simulink model "nn_gensim"  (R2016a)
settings: Solver=VariableStepAuto  StartTime=0.0  StopTime=10.0  RelTol=1e-3
libraries: neural x66
(part 2 of 2)

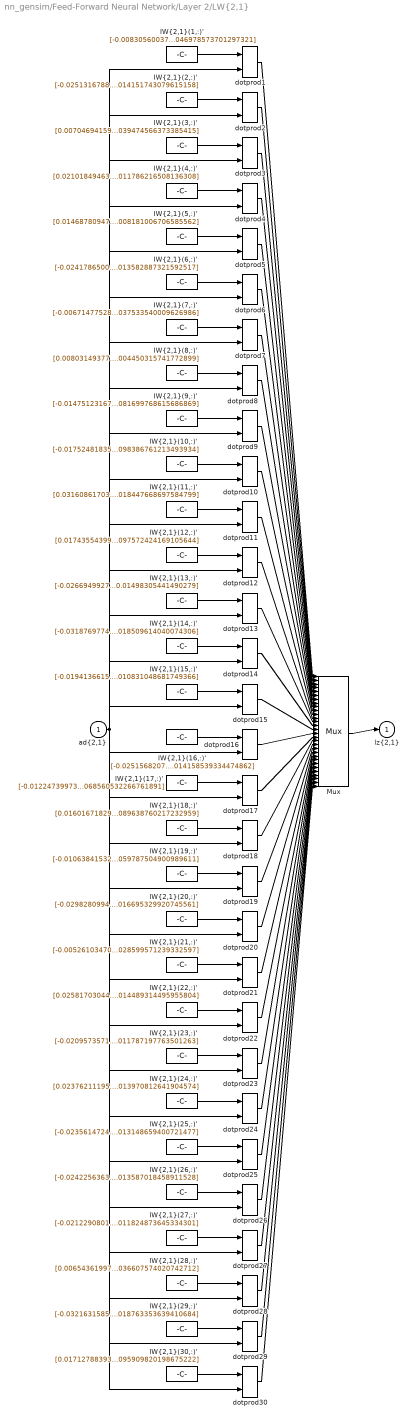
== system nn_gensim/Feed-Forward Neural Network/Layer 2/LW{2,1} ==
  "ad{2,1}" : Inport  PortDimensions=30
      mask Display: e = 0.06;c1 = [120 230 180]/255;c2 = ([120 230 180]+0)/(256+128);c3 = ([120 230 180]+128)/(256+128);patch([0 1 1 0],[0 0 1 1],c1);patch([0 1 1 1-e 1-e 0+e],[0 0 1 1-e 0+e 0+e],c2);patch([0 0 1 1-e 0+e 0+e],[0 1 1 1-e 1-e 0+e],c3);plot([0 1 1 0 0],[0 0 1 1 0]);
  "IW{2,1}(1,:)'" : Constant  Value=[-0.0083056003756890144;0.019113962537947015;-0.0089497074294720546;-0.0098923334864796566;-0.023988299220988073;-0.0018485816845016079;-0.0059618452261974968;0.0069988362336697064;0.036667021342056919;0.016526862034832963;0.030193069855730826;-0.0047630507834777354;-0.018046869018482389;-0.0057026826950931355;0.037752079200427259;0.016557695091664312;0.013106033602432574;-0.019925230456181005;0.039680560899078204;0.025432917279803999;0.00072297603107219274;-0.019455142955335462;-0.01509695277684032;-0.013561420755406835;-0.00075464259463946162;-0.017391870248462917;0.010751916691427063;-0.0050629731985845586;-0.00071487359349162725;-0.0046978573701297321]
      mask Display: e = 0.06;c1 = [120 150 230]/255;c2 = ([120 150 230]+0)/383;c3 = ([120 150 230]+128)/383;patch([0 1 1 0],[0 0 1 1],c1);patch([0 1 1 1-e 1-e 0+e],[0 0 1 1-e 0+e 0+e],c2);patch([0 0 1 1-e 0+e 0+e],[0 1 1 1-e 1-e 0+e],c3);plot([0 1 1 0 0],[0 0 1 1 0]);disp('weights');
  "IW{2,1}(10,:)'" : Constant  Value=[-0.017524818358626806;0.040334814474458656;-0.018584934026375351;-0.020997681047963575;-0.050780548941037972;-0.0034476905494047519;-0.012647174473932836;0.015275522704802792;0.078915212404200449;0.034766129023966738;0.064914340733501982;-0.010010282680391055;-0.038131544108099727;-0.01206243778923099;0.084105228253449155;0.034674216527232619;0.02736829412730514;-0.042075183943914629;0.085704139620146225;0.053900839834691287;0.00099753662040386764;-0.042854177306582489;-0.031996880085286478;-0.028247287853701203;-0.001588847763167444;-0.036339886541172157;0.02264214185105046;-0.01060981341310595;-0.0013587789640045617;-0.0098386761213493934]
      mask Display: e = 0.06;c1 = [120 150 230]/255;c2 = ([120 150 230]+0)/383;c3 = ([120 150 230]+128)/383;patch([0 1 1 0],[0 0 1 1],c1);patch([0 1 1 1-e 1-e 0+e],[0 0 1 1-e 0+e 0+e],c2);patch([0 0 1 1-e 0+e 0+e],[0 1 1 1-e 1-e 0+e],c3);plot([0 1 1 0 0],[0 0 1 1 0]);disp('weights');
  "IW{2,1}(11,:)'" : Constant  Value=[0.031608617033696336;-0.072894856159988572;0.032497541258948992;0.037028062293751475;0.095065968405568177;-0.0025854679662332446;0.022672609607487734;-0.041977003552746424;-0.16800834621404154;-0.060763296536032602;-0.12889957814084452;0.017891408952875096;0.06899010013800265;0.021490887029687971;-0.19237659860623346;-0.059468024825016903;-0.047814292076542045;0.075198049752529444;-0.1858796335369855;-0.10190145864029221;0.0063443741930746611;0.10313747460923257;0.054986646969208179;0.047198965962547634;0.0029349224226672445;0.064302452214189551;-0.041238190569702141;0.019490075273115491;-0.00079340138722999178;0.018447668697584799]
      mask Display: e = 0.06;c1 = [120 150 230]/255;c2 = ([120 150 230]+0)/383;c3 = ([120 150 230]+128)/383;patch([0 1 1 0],[0 0 1 1],c1);patch([0 1 1 1-e 1-e 0+e],[0 0 1 1-e 0+e 0+e],c2);patch([0 0 1 1-e 0+e 0+e],[0 1 1 1-e 1-e 0+e],c3);plot([0 1 1 0 0],[0 0 1 1 0]);disp('weights');
  "IW{2,1}(12,:)'" : Constant  Value=[0.017435543996330929;-0.040142341143420017;0.018474701322763559;0.020931966839192878;0.050465323426277402;0.0034269848078252287;0.012633810047245017;-0.015119790757508161;-0.078491892194480786;-0.034614559781884137;-0.064676958157261766;0.0099795662119423305;0.037936781443958942;0.01201366890879701;-0.083827652877886474;-0.034520744867777162;-0.027203928877341771;0.041896869180871113;-0.085215347287222645;-0.053599186633662151;-0.00091781479818617848;0.042664029462400249;0.031885742582713816;0.028118222040869573;0.0016132091520745346;0.036122832809355798;-0.022546412528904554;0.010549377908676376;0.0013479033309776211;0.0097572424169105644]
      mask Display: e = 0.06;c1 = [120 150 230]/255;c2 = ([120 150 230]+0)/383;c3 = ([120 150 230]+128)/383;patch([0 1 1 0],[0 0 1 1],c1);patch([0 1 1 1-e 1-e 0+e],[0 0 1 1-e 0+e 0+e],c2);patch([0 0 1 1-e 0+e 0+e],[0 1 1 1-e 1-e 0+e],c3);plot([0 1 1 0 0],[0 0 1 1 0]);disp('weights');
  "IW{2,1}(13,:)'" : Constant  Value=[-0.026694992742945192;0.061612330161735056;-0.027653274803672748;-0.03209017288048447;-0.078339461809738109;-0.0032984920599325039;-0.019280886778573432;0.026125586559889606;0.12672985074381135;0.05254292205453958;0.1028317373080775;-0.015138719899045418;-0.058465378962648439;-0.018410447742282243;0.1426089569060506;0.052051523127150716;0.04105910843020593;-0.064224935000000025;0.138707895630444;0.08350353784434883;-0.00030259207296238805;-0.07217030681977768;-0.048668504265280944;-0.041978413631100872;-0.0024148634335991151;-0.054664063752061842;0.034457407503966898;-0.016116981449881235;-0.0014601988631814827;-0.01498305441490279]
      mask Display: e = 0.06;c1 = [120 150 230]/255;c2 = ([120 150 230]+0)/383;c3 = ([120 150 230]+128)/383;patch([0 1 1 0],[0 0 1 1],c1);patch([0 1 1 1-e 1-e 0+e],[0 0 1 1-e 0+e 0+e],c2);patch([0 0 1 1-e 0+e 0+e],[0 1 1 1-e 1-e 0+e],c3);plot([0 1 1 0 0],[0 0 1 1 0]);disp('weights');
  "IW{2,1}(14,:)'" : Constant  Value=[-0.031876977425942685;0.073285499375244853;-0.032295188882699936;-0.037736257112251752;-0.095092447058463245;0.0019240694986817509;-0.022816584395266189;0.040823302705698998;0.16712898248422273;0.060936001349780548;0.12924032585515743;-0.018092945230880942;-0.0694696033517158;-0.021829863852450747;0.19349763967940106;0.059401581781717866;0.047644816424967033;-0.075452140330637518;0.18487501046910346;0.10189553984576843;-0.0055389784205687204;-0.10212528536332899;-0.055994220935609171;-0.047221755005684672;-0.0027621280402611013;-0.064064251531706889;0.041262423698454148;-0.019555242969875469;0.00034805824680751067;-0.018509614040074306]
      mask Display: e = 0.06;c1 = [120 150 230]/255;c2 = ([120 150 230]+0)/383;c3 = ([120 150 230]+128)/383;patch([0 1 1 0],[0 0 1 1],c1);patch([0 1 1 1-e 1-e 0+e],[0 0 1 1-e 0+e 0+e],c2);patch([0 0 1 1-e 0+e 0+e],[0 1 1 1-e 1-e 0+e],c3);plot([0 1 1 0 0],[0 0 1 1 0]);disp('weights');
  "IW{2,1}(15,:)'" : Constant  Value=[-0.019413661578074042;0.044673634539894612;-0.020394867098211009;-0.023348838301773287;-0.056280148408457936;-0.0036788192590742575;-0.014022602890496248;0.017013476590978686;0.087887652471076952;0.038469248573656904;0.072368779142843398;-0.01104288846513549;-0.042281634449772523;-0.013408340227602867;0.095064024539261799;0.038256301227484087;0.030197680839771299;-0.046633071114016482;0.095560722206547571;0.059748872737462252;0.00094440913626948127;-0.048078919304247077;-0.035576359111311552;-0.03112221349266709;-0.001759051666175712;-0.040014263931521771;0.02503986639519926;-0.011699415523057108;-0.0014869690523505858;-0.010831048681749366]
      mask Display: e = 0.06;c1 = [120 150 230]/255;c2 = ([120 150 230]+0)/383;c3 = ([120 150 230]+128)/383;patch([0 1 1 0],[0 0 1 1],c1);patch([0 1 1 1-e 1-e 0+e],[0 0 1 1-e 0+e 0+e],c2);patch([0 0 1 1-e 0+e 0+e],[0 1 1 1-e 1-e 0+e],c3);plot([0 1 1 0 0],[0 0 1 1 0]);disp('weights');
  "IW{2,1}(16,:)'" : Constant  Value=[-0.025156820762488812;0.058054864823515406;-0.026285771892358287;-0.030135766697962155;-0.07372207896226575;-0.0035299672975230914;-0.018137154510463622;0.024068706733688303;0.11810435438225787;0.049635282688275252;0.096016394365898067;-0.014297786003962377;-0.055031126626081464;-0.017324995205387869;0.13096192576822438;0.049293312669310675;0.038919995798569043;-0.060537583862931295;0.12902008870295195;0.078503634724906179;0.00015316680518558015;-0.066545084343001201;-0.045798026988823459;-0.039861832421604487;-0.0022706725238052826;-0.051790823923458386;0.032500592282799695;-0.015220631342250126;-0.0014891042201920946;-0.014158539334474862]
      mask Display: e = 0.06;c1 = [120 150 230]/255;c2 = ([120 150 230]+0)/383;c3 = ([120 150 230]+128)/383;patch([0 1 1 0],[0 0 1 1],c1);patch([0 1 1 1-e 1-e 0+e],[0 0 1 1-e 0+e 0+e],c2);patch([0 0 1 1-e 0+e 0+e],[0 1 1 1-e 1-e 0+e],c3);plot([0 1 1 0 0],[0 0 1 1 0]);disp('weights');
  "IW{2,1}(17,:)'" : Constant  Value=[-0.012247399736339371;0.027919990499933035;-0.012881685984824786;-0.014761102739735237;-0.035202180654838627;-0.0020599440676808594;-0.0092005395436944911;0.01026784494460402;0.054044988107072409;0.024280809606050318;0.045604780665558502;-0.0072409854642835796;-0.025763565138581145;-0.0083617914124821079;0.057354941161920615;0.023963357314242883;0.019098248772568278;-0.029312905852297708;0.058703237012118784;0.037261553017416918;-0.00011879595951369313;-0.030340249318019694;-0.021922420158630104;-0.019631654686126151;-0.0011467033487244838;-0.025190848664596553;0.01592168819718754;-0.0073451151076129048;-0.00076660901977389348;-0.0068560532266761891]
      mask Display: e = 0.06;c1 = [120 150 230]/255;c2 = ([120 150 230]+0)/383;c3 = ([120 150 230]+128)/383;patch([0 1 1 0],[0 0 1 1],c1);patch([0 1 1 1-e 1-e 0+e],[0 0 1 1-e 0+e 0+e],c2);patch([0 0 1 1-e 0+e 0+e],[0 1 1 1-e 1-e 0+e],c3);plot([0 1 1 0 0],[0 0 1 1 0]);disp('weights');
  "IW{2,1}(18,:)'" : Constant  Value=[0.016016718299844059;-0.036819677257688907;0.016932826733152981;0.019256614117186842;0.046276330148802114;0.003265733002481285;0.011585947338575686;-0.01367384074300506;-0.071631228059596111;-0.031788231247260455;-0.059152911619353397;0.0091673768441666373;0.034827598592542565;0.011047247340491433;-0.076308269056356681;-0.031635740099447286;-0.024987921048669898;0.038428093395404941;-0.077738063795936438;-0.049093342238729569;-0.0010158592892138042;0.038752172057827883;0.02933502116447145;0.025798766205491173;0.0014571105509814965;0.033115494438306838;-0.020678915092600374;0.0096725881977464435;0.0012950684968727408;0.0089638760217232959]
      mask Display: e = 0.06;c1 = [120 150 230]/255;c2 = ([120 150 230]+0)/383;c3 = ([120 150 230]+128)/383;patch([0 1 1 0],[0 0 1 1],c1);patch([0 1 1 1-e 1-e 0+e],[0 0 1 1-e 0+e 0+e],c2);patch([0 0 1 1-e 0+e 0+e],[0 1 1 1-e 1-e 0+e],c3);plot([0 1 1 0 0],[0 0 1 1 0]);disp('weights');
  "IW{2,1}(19,:)'" : Constant  Value=[-0.010638415324202181;0.024466298045185055;-0.011374419942669347;-0.012723305433966443;-0.030681304419064404;-0.0023319126550419996;-0.0076728073988347797;0.008935450570325347;0.047047539700759283;0.021140029180016316;0.038844367396343012;-0.0061025300069295308;-0.02310580991056229;-0.0073129602516543556;0.049017418731317368;0.021123843026066708;0.01670017628268463;-0.025510370721981802;0.050960130024091943;0.032517967654103405;0.00085817745947512928;-0.025095581533722718;-0.019419310619989381;-0.017271705252226679;-0.00097288260425591332;-0.022146740960695875;0.013749697048640411;-0.006447833518349144;-0.00090654148627930954;-0.0059787504900989611]
      mask Display: e = 0.06;c1 = [120 150 230]/255;c2 = ([120 150 230]+0)/383;c3 = ([120 150 230]+128)/383;patch([0 1 1 0],[0 0 1 1],c1);patch([0 1 1 1-e 1-e 0+e],[0 0 1 1-e 0+e 0+e],c2);patch([0 0 1 1-e 0+e 0+e],[0 1 1 1-e 1-e 0+e],c3);plot([0 1 1 0 0],[0 0 1 1 0]);disp('weights');
  "IW{2,1}(2,:)'" : Constant  Value=[-0.025131678864987378;0.058073066887020866;-0.026304061314684563;-0.030104242994924962;-0.073779720571755469;-0.0034981920824001225;-0.01812939659958078;0.024156378833896888;0.11821593497827068;0.049663313648724436;0.096042124009199092;-0.014294642763133273;-0.05503717759726675;-0.017307544324334762;0.13095369921667074;0.04934996437657814;0.038951372167574473;-0.060539636418673493;0.12915357970896532;0.078553239139516437;9.3957580113377347e-05;-0.066626496446194422;-0.045745316794285992;-0.039898573968896484;-0.0022783639220442416;-0.05185149241761703;0.032521618965200123;-0.015226527221287534;-0.0014598757765509882;-0.014151743079615158]
      mask Display: e = 0.06;c1 = [120 150 230]/255;c2 = ([120 150 230]+0)/383;c3 = ([120 150 230]+128)/383;patch([0 1 1 0],[0 0 1 1],c1);patch([0 1 1 1-e 1-e 0+e],[0 0 1 1-e 0+e 0+e],c2);patch([0 0 1 1-e 0+e 0+e],[0 1 1 1-e 1-e 0+e],c3);plot([0 1 1 0 0],[0 0 1 1 0]);disp('weights');
  "IW{2,1}(20,:)'" : Constant  Value=[-0.029828099428775366;0.068669778965433789;-0.030418611782497933;-0.035436710105212668;-0.088756277463647185;-0.0016946136484623331;-0.021317691930237283;0.032650862920382877;0.14691496644874313;0.058345195184973837;0.11773707030965279;-0.016112646226604084;-0.064583241860201798;-0.020487702029837157;0.16994777149515553;0.057554595379670795;0.046089238996385264;-0.071775931966892151;0.16215608604950973;0.094404691817460015;-0.0027083072941593363;-0.086134883721040681;-0.053278245086398092;-0.046227102422427092;-0.0027190071723236352;-0.060835780095390792;0.038472042278304863;-0.017728882539972443;-0.0010997381241217134;-0.016695329920745561]
      mask Display: e = 0.06;c1 = [120 150 230]/255;c2 = ([120 150 230]+0)/383;c3 = ([120 150 230]+128)/383;patch([0 1 1 0],[0 0 1 1],c1);patch([0 1 1 1-e 1-e 0+e],[0 0 1 1-e 0+e 0+e],c2);patch([0 0 1 1-e 0+e 0+e],[0 1 1 1-e 1-e 0+e],c3);plot([0 1 1 0 0],[0 0 1 1 0]);disp('weights');
  "IW{2,1}(21,:)'" : Constant  Value=[-0.0052610347081779663;0.011997340944229136;-0.0054199539471969536;-0.0064301647679833839;-0.014965417534536252;-0.0012031196345792009;-0.0038298933070947156;0.0041350288513638377;0.022886690125965684;0.01040506983314101;0.01920305344715776;-0.0029587945971189383;-0.011366498206918286;-0.0036769412168634525;0.024553087182836029;0.010273861739478729;0.0081335729662590974;-0.012536155939624923;0.024774679008191011;0.015823004227201544;0.00042560970528744181;-0.012214264761215954;-0.0097789605437299202;-0.0083946276078156971;-0.00047986162826767816;-0.010655406049252452;0.0067481108040413169;-0.003120167698468723;-0.00051113328768417671;-0.0028599571239332597]
      mask Display: e = 0.06;c1 = [120 150 230]/255;c2 = ([120 150 230]+0)/383;c3 = ([120 150 230]+128)/383;patch([0 1 1 0],[0 0 1 1],c1);patch([0 1 1 1-e 1-e 0+e],[0 0 1 1-e 0+e 0+e],c2);patch([0 0 1 1-e 0+e 0+e],[0 1 1 1-e 1-e 0+e],c3);plot([0 1 1 0 0],[0 0 1 1 0]);disp('weights');
  "IW{2,1}(22,:)'" : Constant  Value=[0.025817030444396732;-0.059676414292279926;0.026972559641166287;0.030996433947275505;0.075829409120873464;0.0033676180025425753;0.018687674597139881;-0.025109768314917888;-0.12211737594324765;-0.051038346647778086;-0.099189138221123768;0.014653149811589883;0.056492088416734941;0.017809070916579083;-0.13619609291936915;-0.050714586123944604;-0.03996347892590834;0.062272435635577404;-0.13350994222697937;-0.080808693568826903;0.0003503470366280497;0.06920672592789788;0.046973850143169682;0.040904226721356816;0.0023901239221090827;0.053167301718389522;-0.033421673703184399;0.015618985557533107;0.0014161691257629902;0.014489314495955804]
      mask Display: e = 0.06;c1 = [120 150 230]/255;c2 = ([120 150 230]+0)/383;c3 = ([120 150 230]+128)/383;patch([0 1 1 0],[0 0 1 1],c1);patch([0 1 1 1-e 1-e 0+e],[0 0 1 1-e 0+e 0+e],c2);patch([0 0 1 1-e 0+e 0+e],[0 1 1 1-e 1-e 0+e],c3);plot([0 1 1 0 0],[0 0 1 1 0]);disp('weights');
  "IW{2,1}(23,:)'" : Constant  Value=[-0.020957357151804693;0.048347300677523547;-0.022145982680321339;-0.025094837318185667;-0.061072110227237603;-0.0037096475108920482;-0.015118124608381011;0.01892634613601387;0.095934363233959527;0.04155952825480963;0.07854720933485107;-0.01195886294338698;-0.045747499657605092;-0.014418386120638548;0.10367367481569201;0.041408692771618738;0.032678811232905586;-0.050431230717510545;0.10440151965585052;0.064920425919154159;0.0008169472865166168;-0.052797769437693709;-0.038225650942368877;-0.033635478492212142;-0.0019041270880817815;-0.043446467242873182;0.02711014467296597;-0.012704548682364921;-0.0014752275551377025;-0.011787197763501263]
      mask Display: e = 0.06;c1 = [120 150 230]/255;c2 = ([120 150 230]+0)/383;c3 = ([120 150 230]+128)/383;patch([0 1 1 0],[0 0 1 1],c1);patch([0 1 1 1-e 1-e 0+e],[0 0 1 1-e 0+e 0+e],c2);patch([0 0 1 1-e 0+e 0+e],[0 1 1 1-e 1-e 0+e],c3);plot([0 1 1 0 0],[0 0 1 1 0]);disp('weights');
  "IW{2,1}(24,:)'" : Constant  Value=[0.023762111957027158;-0.050414631997961187;0.023966063330787629;0.026414804515273227;0.069397155774670011;-0.0019037275139693927;0.017269861052220167;-0.025318918943734784;-0.1047272722851622;-0.045143706114235918;-0.092318758662667297;0.011849349130237359;0.039347876974872825;0.016200937256073404;-0.11546694159844476;-0.043035748004879623;-0.038048762268926381;0.054781195240020217;-0.11882665560186687;-0.072591152338108825;0.010269411233009356;0.067869028797714753;0.03330076286145079;0.035548673612533811;0.0017591441582085752;0.048488960326691984;-0.03130980499604729;0.013813376195273591;-0.00042699096728539694;0.013970812641904574]
      mask Display: e = 0.06;c1 = [120 150 230]/255;c2 = ([120 150 230]+0)/383;c3 = ([120 150 230]+128)/383;patch([0 1 1 0],[0 0 1 1],c1);patch([0 1 1 1-e 1-e 0+e],[0 0 1 1-e 0+e 0+e],c2);patch([0 0 1 1-e 0+e 0+e],[0 1 1 1-e 1-e 0+e],c3);plot([0 1 1 0 0],[0 0 1 1 0]);disp('weights');
  "IW{2,1}(25,:)'" : Constant  Value=[-0.023561472421982713;0.054331752038774071;-0.024529872825749664;-0.028372962550169432;-0.068759666737134614;-0.0037915702172108784;-0.017035063653915633;0.021673804891123707;0.1090501774627913;0.046575749112541351;0.089301929980748748;-0.013368586222116605;-0.051524505279527677;-0.016273157830019973;0.12061047575315614;0.046221945145444511;0.036475014912460364;-0.056694904730814809;0.11894361480681187;0.073088829187946514;0.00057413351736356638;-0.060853811586294097;-0.043185260633266685;-0.03743910178308299;-0.0021400907381204808;-0.048382107064453179;0.030401025549228165;-0.014178081320290048;-0.0015822012464757509;-0.013148659400721477]
      mask Display: e = 0.06;c1 = [120 150 230]/255;c2 = ([120 150 230]+0)/383;c3 = ([120 150 230]+128)/383;patch([0 1 1 0],[0 0 1 1],c1);patch([0 1 1 1-e 1-e 0+e],[0 0 1 1-e 0+e 0+e],c2);patch([0 0 1 1-e 0+e 0+e],[0 1 1 1-e 1-e 0+e],c3);plot([0 1 1 0 0],[0 0 1 1 0]);disp('weights');
  "IW{2,1}(26,:)'" : Constant  Value=[-0.024225636316209963;0.055921583307778938;-0.025348764190545357;-0.029051101370178724;-0.070922867884940913;-0.0036523765095095311;-0.017499172972537544;0.022822410383101566;0.11301792723806638;0.047913166473140749;0.092129586256700965;-0.013761041893200918;-0.052977306621000565;-0.016684366316797469;0.12475807695957174;0.047613088926130004;0.037578716433856699;-0.058345621216225489;0.12335135826948916;0.075460805937169848;0.00030516629717828166;-0.063324555886756409;-0.044178644238480932;-0.038534818977491281;-0.0022171384982168254;-0.049940190130057044;0.031323631932409987;-0.014641769778095835;-0.0014934854154008649;-0.013587018458911528]
      mask Display: e = 0.06;c1 = [120 150 230]/255;c2 = ([120 150 230]+0)/383;c3 = ([120 150 230]+128)/383;patch([0 1 1 0],[0 0 1 1],c1);patch([0 1 1 1-e 1-e 0+e],[0 0 1 1-e 0+e 0+e],c2);patch([0 0 1 1-e 0+e 0+e],[0 1 1 1-e 1-e 0+e],c3);plot([0 1 1 0 0],[0 0 1 1 0]);disp('weights');
  "IW{2,1}(27,:)'" : Constant  Value=[-0.021229080197496739;0.048857449734420681;-0.022209497208424016;-0.025563213084126735;-0.061640129584370741;-0.0038023067180208256;-0.015341060841718004;0.018888355549275038;0.096846741599454084;0.042002787978543406;0.079642268412609046;-0.012048671890145631;-0.046270485617316316;-0.014667799223781591;0.10582567571694941;0.041758372060170981;0.032938810279003639;-0.051011123533214603;0.10544601870384707;0.06550192309925551;0.00078444332507273621;-0.053398391642060776;-0.038898659970153605;-0.033893663168247073;-0.0019230779917130442;-0.043654377394106804;0.027371655366959447;-0.012788380344298984;-0.0015808524825874049;-0.011824873645334301]
      mask Display: e = 0.06;c1 = [120 150 230]/255;c2 = ([120 150 230]+0)/383;c3 = ([120 150 230]+128)/383;patch([0 1 1 0],[0 0 1 1],c1);patch([0 1 1 1-e 1-e 0+e],[0 0 1 1-e 0+e 0+e],c2);patch([0 0 1 1-e 0+e 0+e],[0 1 1 1-e 1-e 0+e],c3);plot([0 1 1 0 0],[0 0 1 1 0]);disp('weights');
  "IW{2,1}(28,:)'" : Constant  Value=[0.0065436199750688673;-0.015027504953591843;0.006974625573801841;0.0078538285071269136;0.018805371950142893;0.0014771166752703363;0.0047291408283852438;-0.0053985439816228121;-0.028728965940826964;-0.013005793419592841;-0.023796907117119563;0.0037490994392130744;0.014189596448692315;0.0045161886969702567;-0.029868343825695622;-0.012967990812818499;-0.010259095812471076;0.015663155351010323;-0.031093069307081573;-0.01991723007190491;-0.00055937457249222991;0.015243706568819234;0.011978693823600964;0.010629868728769407;0.0005994675380060193;0.013590588657373651;-0.0084577858758005213;0.0039585830368520682;0.00057501330107201192;0.0036607574020742712]
      mask Display: e = 0.06;c1 = [120 150 230]/255;c2 = ([120 150 230]+0)/383;c3 = ([120 150 230]+128)/383;patch([0 1 1 0],[0 0 1 1],c1);patch([0 1 1 1-e 1-e 0+e],[0 0 1 1-e 0+e 0+e],c2);patch([0 0 1 1-e 0+e 0+e],[0 1 1 1-e 1-e 0+e],c3);plot([0 1 1 0 0],[0 0 1 1 0]);disp('weights');
  "IW{2,1}(29,:)'" : Constant  Value=[-0.032163158533931008;0.074117828768836588;-0.032763433958060285;-0.037439426383892548;-0.097306914691076413;0.00425862308813917;-0.023072670047185558;0.045535809746374667;0.17519667574004533;0.061530999134061196;0.13299100893861082;-0.017990053763580718;-0.069914692609739884;-0.021801914306939851;0.20209377655542732;0.059834330508469348;0.048612196495728267;-0.076327089002449847;0.19435267313951909;0.10422496523945289;-0.0081896718674689742;-0.10926645673909779;-0.055366306614678465;-0.047324235295989787;-0.0030926495529430952;-0.065096411623604758;0.04205947945273053;-0.019722535184827601;0.0014420751755535536;-0.018763353639410684]
      mask Display: e = 0.06;c1 = [120 150 230]/255;c2 = ([120 150 230]+0)/383;c3 = ([120 150 230]+128)/383;patch([0 1 1 0],[0 0 1 1],c1);patch([0 1 1 1-e 1-e 0+e],[0 0 1 1-e 0+e 0+e],c2);patch([0 0 1 1-e 0+e 0+e],[0 1 1 1-e 1-e 0+e],c3);plot([0 1 1 0 0],[0 0 1 1 0]);disp('weights');
  "IW{2,1}(3,:)'" : Constant  Value=[0.0070469415910385282;-0.016177436634165147;0.0075008917049772666;0.0084561191101651199;0.020259537709289177;0.0015969459932051522;0.0050848315963186704;-0.0058253459799596152;-0.030975638329399771;-0.014004901187448909;-0.025648940344488384;0.0040313728741193282;0.015288332869058308;0.0048649988988983001;-0.03223379496049069;-0.013975722744964125;-0.01104916286120673;0.01687817610555966;-0.033507375347502609;-0.021465055444343149;-0.00061197938068524409;0.016448695291971717;0.012896984831575423;0.011437414626064492;0.0006369384776121499;0.014622800838986047;-0.0091087839869899052;0.0042590142297167771;0.0006292176952032313;0.0039474566373385415]
      mask Display: e = 0.06;c1 = [120 150 230]/255;c2 = ([120 150 230]+0)/383;c3 = ([120 150 230]+128)/383;patch([0 1 1 0],[0 0 1 1],c1);patch([0 1 1 1-e 1-e 0+e],[0 0 1 1-e 0+e 0+e],c2);patch([0 0 1 1-e 0+e 0+e],[0 1 1 1-e 1-e 0+e],c3);plot([0 1 1 0 0],[0 0 1 1 0]);disp('weights');
  "IW{2,1}(30,:)'" : Constant  Value=[0.01712788393662381;-0.039410293072330585;0.018108005486710078;0.020584813608518014;0.049543736262955877;0.0034188416731501209;0.012373519176772908;-0.014777390346386317;-0.076940069114085421;-0.033973650048574257;-0.063435652333261539;0.0097673697651435559;0.037274005378839258;0.011811156013551025;-0.082225877650525511;-0.03385441463117423;-0.026710388238390594;0.041118373464316051;-0.083531721718123952;-0.052590899401517635;-0.0010192798861558851;0.041740385111230183;0.03135938987485816;0.027590443862758302;0.0015597984700660369;0.035427254259479277;-0.022112899234676919;0.010354205041791938;0.001373264726472419;0.0095909820198675222]
      mask Display: e = 0.06;c1 = [120 150 230]/255;c2 = ([120 150 230]+0)/383;c3 = ([120 150 230]+128)/383;patch([0 1 1 0],[0 0 1 1],c1);patch([0 1 1 1-e 1-e 0+e],[0 0 1 1-e 0+e 0+e],c2);patch([0 0 1 1-e 0+e 0+e],[0 1 1 1-e 1-e 0+e],c3);plot([0 1 1 0 0],[0 0 1 1 0]);disp('weights');
  "IW{2,1}(4,:)'" : Constant  Value=[0.021018494639008137;-0.048422364950132087;0.022120225602499072;0.025218595365931726;0.06113598143777603;0.0037340968260247479;0.015162852770423636;-0.018857451273304029;-0.096010106678520224;-0.041615303205548883;-0.078760267641770576;0.011963229891929274;0.045834304304471427;0.014484884029716708;-0.10420805537396845;-0.041441493635766061;-0.032705972013988296;0.050526067781640267;-0.10452334187295746;-0.064970888705483343;-0.00082591038262757081;0.052877238417294595;0.03839864378174606;0.033656112908710817;0.0019071998617308146;0.04342612791052148;-0.027142505893598488;0.012711381722292652;0.0015203690435733261;0.011786216508136308]
      mask Display: e = 0.06;c1 = [120 150 230]/255;c2 = ([120 150 230]+0)/383;c3 = ([120 150 230]+128)/383;patch([0 1 1 0],[0 0 1 1],c1);patch([0 1 1 1-e 1-e 0+e],[0 0 1 1-e 0+e 0+e],c2);patch([0 0 1 1-e 0+e 0+e],[0 1 1 1-e 1-e 0+e],c3);plot([0 1 1 0 0],[0 0 1 1 0]);disp('weights');
  "IW{2,1}(5,:)'" : Constant  Value=[0.014687809471947651;-0.033761041948008934;0.015495704902200244;0.017689879660476214;0.04239217072469123;0.0030766794340142006;0.010636908063930185;-0.012418147588878596;-0.065444525294683309;-0.029151820386824904;-0.054138345998576407;0.008364542619664312;0.03193210977506479;0.010144649850732967;-0.069646230617862723;-0.029016134859478265;-0.022946675511865487;0.035232946980147721;-0.070989995915150914;-0.044931414289357596;-0.00099571460969854336;0.035272306157751683;0.0269634487011014;0.023685734525732301;0.0013351047079472539;0.030325307846787265;-0.01895786437117776;0.0088559578500785694;0.0012289942006464161;0.008181006706585562]
      mask Display: e = 0.06;c1 = [120 150 230]/255;c2 = ([120 150 230]+0)/383;c3 = ([120 150 230]+128)/383;patch([0 1 1 0],[0 0 1 1],c1);patch([0 1 1 1-e 1-e 0+e],[0 0 1 1-e 0+e 0+e],c2);patch([0 0 1 1-e 0+e 0+e],[0 1 1 1-e 1-e 0+e],c3);plot([0 1 1 0 0],[0 0 1 1 0]);disp('weights');
  "IW{2,1}(6,:)'" : Constant  Value=[-0.024178650038271625;0.055849244854547321;-0.025351731079285796;-0.028977550377926105;-0.070833016988131423;-0.0036382474595448486;-0.017468108684774206;0.022812902465132737;0.11287279874971068;0.047836295974878026;0.09193697446513871;-0.013769667003876055;-0.05291482847648632;-0.016636451840627241;0.12438288058655883;0.04754401730281739;0.037535637277431873;-0.058252753133732356;0.12319681325896514;0.075366310980345824;0.00035550833661809227;-0.0632254095743989;-0.044092679658967397;-0.038481752047552026;-0.0022142467405009457;-0.049913714533790642;0.031279951602395002;-0.014635523432089809;-0.0014766168692462599;-0.013582887321592517]
      mask Display: e = 0.06;c1 = [120 150 230]/255;c2 = ([120 150 230]+0)/383;c3 = ([120 150 230]+128)/383;patch([0 1 1 0],[0 0 1 1],c1);patch([0 1 1 1-e 1-e 0+e],[0 0 1 1-e 0+e 0+e],c2);patch([0 0 1 1-e 0+e 0+e],[0 1 1 1-e 1-e 0+e],c3);plot([0 1 1 0 0],[0 0 1 1 0]);disp('weights');
  "IW{2,1}(7,:)'" : Constant  Value=[-0.006714775285058568;0.015425366990594375;-0.0071444372367655837;-0.008075304859312047;-0.019301518112276747;-0.0015215697292773258;-0.004863276218779581;0.005525966017705072;0.029489997543609439;0.013342060933059506;0.024446416592565034;-0.0038477265564835971;-0.014570887565618196;-0.0046396811118881278;0.030748154307727864;0.013301458245725057;0.01053020966166706;-0.016076184054737482;0.031906115183904064;0.020429476791613103;0.00056497788477697503;-0.015657172991457212;-0.012317461913503998;-0.010891398828204035;-0.00061294385475724352;-0.013920619008982459;0.0086725741061264242;-0.0040642753947364458;-0.00059209670490314298;-0.0037533540009626986]
      mask Display: e = 0.06;c1 = [120 150 230]/255;c2 = ([120 150 230]+0)/383;c3 = ([120 150 230]+128)/383;patch([0 1 1 0],[0 0 1 1],c1);patch([0 1 1 1-e 1-e 0+e],[0 0 1 1-e 0+e 0+e],c2);patch([0 0 1 1-e 0+e 0+e],[0 1 1 1-e 1-e 0+e],c3);plot([0 1 1 0 0],[0 0 1 1 0]);disp('weights');
  "IW{2,1}(8,:)'" : Constant  Value=[0.0080314937761839737;-0.018379039304677894;0.0084465819186563956;0.0096925062283603688;0.022978722961638005;0.0018118591537378951;0.0058166061534915608;-0.0065338269066266969;-0.035185528077176745;-0.015916713400994962;-0.029276226802080352;0.0045674097406264652;0.017380680440984175;0.0055569016880365352;-0.037107605242382539;-0.015819044037708299;-0.012500762097102065;0.019189587280132241;-0.038087091699989355;-0.024330222312929192;-0.00065076971668176714;0.018746731365779805;0.014768481516352853;0.012939161004535224;0.00073118410427518328;0.016496981311702973;-0.010329789055239461;0.0048269109447742859;0.00073056531980228445;0.004450315741772899]
      mask Display: e = 0.06;c1 = [120 150 230]/255;c2 = ([120 150 230]+0)/383;c3 = ([120 150 230]+128)/383;patch([0 1 1 0],[0 0 1 1],c1);patch([0 1 1 1-e 1-e 0+e],[0 0 1 1-e 0+e 0+e],c2);patch([0 0 1 1-e 0+e 0+e],[0 1 1 1-e 1-e 0+e],c3);plot([0 1 1 0 0],[0 0 1 1 0]);disp('weights');
  "IW{2,1}(9,:)'" : Constant  Value=[-0.014751231675251003;0.033858211664294161;-0.015469065080710477;-0.017815759974031453;-0.04243324459776264;-0.0031081511070360454;-0.010686728797206908;0.012333044238216585;0.065555558178400627;0.029243533798472644;0.054359878779857408;-0.0083997244222791638;-0.032030021512147198;-0.010208504191575235;0.070141345388912757;0.029057507322596623;0.022946024870107325;-0.035335075106669243;0.071113496446445448;0.044992891708354681;0.00098078285727177107;-0.035363952703147052;-0.027130858993164534;-0.023705472162509202;-0.001349940174421647;-0.030304079215602193;0.019010605988897811;-0.0088608495951366679;-0.0012656783586346809;-0.0081699768615686869]
      mask Display: e = 0.06;c1 = [120 150 230]/255;c2 = ([120 150 230]+0)/383;c3 = ([120 150 230]+128)/383;patch([0 1 1 0],[0 0 1 1],c1);patch([0 1 1 1-e 1-e 0+e],[0 0 1 1-e 0+e 0+e],c2);patch([0 0 1 1-e 0+e 0+e],[0 1 1 1-e 1-e 0+e],c3);plot([0 1 1 0 0],[0 0 1 1 0]);disp('weights');
  Mux : Mux  Inputs=30
      mask Display: e = 0.06;c1 = [120 150 230]/255;c2 = ([120 150 230]+0)/383;c3 = ([120 150 230]+128)/383;patch([0 1 1 0],[0 0 1 1],c1);patch([0 1 1 1-e 1-e 0+e],[0 0 1 1-e 0+e 0+e],c2);patch([0 0 1 1-e 0+e 0+e],[0 1 1 1-e 1-e 0+e],c3);plot([0 1 1 0 0],[0 0 1 1 0]);disp('Mux');
  dotprod{1..30} (30 alike) : neural/Weight Functions/dotprod
  "lz{2,1}" : Outport
      mask Display: e = 0.06;c1 = [120 230 180]/255;c2 = ([120 230 180]+0)/(256+128);c3 = ([120 230 180]+128)/(256+128);patch([0 1 1 0],[0 0 1 1],c1);patch([0 1 1 1-e 1-e 0+e],[0 0 1 1-e 0+e 0+e],c2);patch([0 0 1 1-e 0+e 0+e],[0 1 1 1-e 1-e 0+e],c3);plot([0 1 1 0 0],[0 0 1 1 0]);
  wires:
  "IW{2,1}(1,:)'"/1 -> dotprod1/1
  "ad{2,1}"/1 -> dotprod1/2, dotprod2/2, dotprod3/2, dotprod4/2, dotprod5/2, dotprod6/2, dotprod7/2, dotprod8/2, dotprod9/2, dotprod10/2, dotprod11/2, dotprod12/2, dotprod13/2, dotprod14/2, dotprod15/2, dotprod16/2, dotprod17/2, dotprod18/2, dotprod19/2, dotprod20/2, dotprod21/2, dotprod22/2, dotprod23/2, dotprod24/2, dotprod25/2, dotprod26/2, dotprod27/2, dotprod28/2, dotprod29/2, dotprod30/2
  dotprod1/1 -> Mux/1
  "IW{2,1}(2,:)'"/1 -> dotprod2/1
  dotprod2/1 -> Mux/2
  "IW{2,1}(3,:)'"/1 -> dotprod3/1
  dotprod3/1 -> Mux/3
  "IW{2,1}(4,:)'"/1 -> dotprod4/1
  dotprod4/1 -> Mux/4
  "IW{2,1}(5,:)'"/1 -> dotprod5/1
  dotprod5/1 -> Mux/5
  "IW{2,1}(6,:)'"/1 -> dotprod6/1
  dotprod6/1 -> Mux/6
  "IW{2,1}(7,:)'"/1 -> dotprod7/1
  dotprod7/1 -> Mux/7
  "IW{2,1}(8,:)'"/1 -> dotprod8/1
  dotprod8/1 -> Mux/8
  "IW{2,1}(9,:)'"/1 -> dotprod9/1
  dotprod9/1 -> Mux/9
  "IW{2,1}(10,:)'"/1 -> dotprod10/1
  dotprod10/1 -> Mux/10
  "IW{2,1}(11,:)'"/1 -> dotprod11/1
  dotprod11/1 -> Mux/11
  "IW{2,1}(12,:)'"/1 -> dotprod12/1
  dotprod12/1 -> Mux/12
  "IW{2,1}(13,:)'"/1 -> dotprod13/1
  dotprod13/1 -> Mux/13
  "IW{2,1}(14,:)'"/1 -> dotprod14/1
  dotprod14/1 -> Mux/14
  "IW{2,1}(15,:)'"/1 -> dotprod15/1
  dotprod15/1 -> Mux/15
  "IW{2,1}(16,:)'"/1 -> dotprod16/1
  dotprod16/1 -> Mux/16
  "IW{2,1}(17,:)'"/1 -> dotprod17/1
  dotprod17/1 -> Mux/17
  "IW{2,1}(18,:)'"/1 -> dotprod18/1
  dotprod18/1 -> Mux/18
  "IW{2,1}(19,:)'"/1 -> dotprod19/1
  dotprod19/1 -> Mux/19
  "IW{2,1}(20,:)'"/1 -> dotprod20/1
  dotprod20/1 -> Mux/20
  "IW{2,1}(21,:)'"/1 -> dotprod21/1
  dotprod21/1 -> Mux/21
  "IW{2,1}(22,:)'"/1 -> dotprod22/1
  dotprod22/1 -> Mux/22
  "IW{2,1}(23,:)'"/1 -> dotprod23/1
  dotprod23/1 -> Mux/23
  "IW{2,1}(24,:)'"/1 -> dotprod24/1
  dotprod24/1 -> Mux/24
  "IW{2,1}(25,:)'"/1 -> dotprod25/1
  dotprod25/1 -> Mux/25
  "IW{2,1}(26,:)'"/1 -> dotprod26/1
  dotprod26/1 -> Mux/26
  "IW{2,1}(27,:)'"/1 -> dotprod27/1
  dotprod27/1 -> Mux/27
  "IW{2,1}(28,:)'"/1 -> dotprod28/1
  dotprod28/1 -> Mux/28
  "IW{2,1}(29,:)'"/1 -> dotprod29/1
  dotprod29/1 -> Mux/29
  "IW{2,1}(30,:)'"/1 -> dotprod30/1
  dotprod30/1 -> Mux/30
  Mux/1 -> "lz{2,1}"/1

== system nn_gensim/Feed-Forward Neural Network/Layer 3/Delays 1 ==
  "p{3}" : Inport  PortDimensions=30
      mask Display: e = 0.06;c1 = [120 230 180]/255;c2 = ([120 230 180]+0)/(256+128);c3 = ([120 230 180]+128)/(256+128);patch([0 1 1 0],[0 0 1 1],c1);patch([0 1 1 1-e 1-e 0+e],[0 0 1 1-e 0+e 0+e],c2);patch([0 0 1 1-e 0+e 0+e],[0 1 1 1-e 1-e 0+e],c3);plot([0 1 1 0 0],[0 0 1 1 0]);
  mux : Mux  Inputs=1
      mask Display: e = 0.06;c1 = [120 150 230]/255;c2 = ([120 150 230]+0)/383;c3 = ([120 150 230]+128)/383;patch([0 1 1 0],[0 0 1 1],c1);patch([0 1 1 1-e 1-e 0+e],[0 0 1 1-e 0+e 0+e],c2);patch([0 0 1 1-e 0+e 0+e],[0 1 1 1-e 1-e 0+e],c3);plot([0 1 1 0 0],[0 0 1 1 0]);disp('Mux')
  "pd{3,2}" : Outport
      mask Display: e = 0.06;c1 = [120 230 180]/255;c2 = ([120 230 180]+0)/(256+128);c3 = ([120 230 180]+128)/(256+128);patch([0 1 1 0],[0 0 1 1],c1);patch([0 1 1 1-e 1-e 0+e],[0 0 1 1-e 0+e 0+e],c2);patch([0 0 1 1-e 0+e 0+e],[0 1 1 1-e 1-e 0+e],c3);plot([0 1 1 0 0],[0 0 1 1 0]);
  wires:
  "p{3}"/1 -> mux/1
  mux/1 -> "pd{3,2}"/1

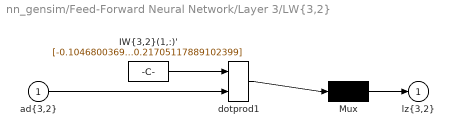
== system nn_gensim/Feed-Forward Neural Network/Layer 3/LW{3,2} ==
  "ad{3,2}" : Inport  PortDimensions=30
      mask Display: e = 0.06;c1 = [120 230 180]/255;c2 = ([120 230 180]+0)/(256+128);c3 = ([120 230 180]+128)/(256+128);patch([0 1 1 0],[0 0 1 1],c1);patch([0 1 1 1-e 1-e 0+e],[0 0 1 1-e 0+e 0+e],c2);patch([0 0 1 1-e 0+e 0+e],[0 1 1 1-e 1-e 0+e],c3);plot([0 1 1 0 0],[0 0 1 1 0]);
  "IW{3,2}(1,:)'" : Constant  Value=[-0.10468003696309827;-0.34269393548702592;0.086534561443418673;0.27369662400452421;0.1826185289046304;-0.32565397361838566;-0.082070491887762387;0.096517298873166429;-0.18132930405090716;-0.22432439218721617;0.51760660165730243;0.22212498096120947;-0.36656922044991719;-0.50909892430145753;-0.24784601874779358;-0.34194788352255379;-0.14938395469661561;0.20150940661242583;-0.13304640233791562;-0.42936199089588428;-0.0603846988423297;0.35312689761657701;-0.27528167465034098;0.30599761734311992;-0.31029873007702502;-0.32520911198113339;-0.27352334677440154;0.080348498618795977;-0.54143422037287148;0.21705117889102399]
      mask Display: e = 0.06;c1 = [120 150 230]/255;c2 = ([120 150 230]+0)/383;c3 = ([120 150 230]+128)/383;patch([0 1 1 0],[0 0 1 1],c1);patch([0 1 1 1-e 1-e 0+e],[0 0 1 1-e 0+e 0+e],c2);patch([0 0 1 1-e 0+e 0+e],[0 1 1 1-e 1-e 0+e],c3);plot([0 1 1 0 0],[0 0 1 1 0]);disp('weights');
  Mux : Mux  Inputs=1
      mask Display: e = 0.06;c1 = [120 150 230]/255;c2 = ([120 150 230]+0)/383;c3 = ([120 150 230]+128)/383;patch([0 1 1 0],[0 0 1 1],c1);patch([0 1 1 1-e 1-e 0+e],[0 0 1 1-e 0+e 0+e],c2);patch([0 0 1 1-e 0+e 0+e],[0 1 1 1-e 1-e 0+e],c3);plot([0 1 1 0 0],[0 0 1 1 0]);disp('Mux');
  dotprod1 : neural/Weight Functions/dotprod
  "lz{3,2}" : Outport
      mask Display: e = 0.06;c1 = [120 230 180]/255;c2 = ([120 230 180]+0)/(256+128);c3 = ([120 230 180]+128)/(256+128);patch([0 1 1 0],[0 0 1 1],c1);patch([0 1 1 1-e 1-e 0+e],[0 0 1 1-e 0+e 0+e],c2);patch([0 0 1 1-e 0+e 0+e],[0 1 1 1-e 1-e 0+e],c3);plot([0 1 1 0 0],[0 0 1 1 0]);
  wires:
  "IW{3,2}(1,:)'"/1 -> dotprod1/1
  "ad{3,2}"/1 -> dotprod1/2
  dotprod1/1 -> Mux/1
  Mux/1 -> "lz{3,2}"/1
